simulink model "test_socket"  (Simulink 7.4)
settings: Solver=ode45  StartTime=0.0  StopTime=15.0  FixedStep=0.01  RelTol=1e-3
libraries: instrumentlib x2
settings Model: Creator=tasora  LastModifiedBy=tasora

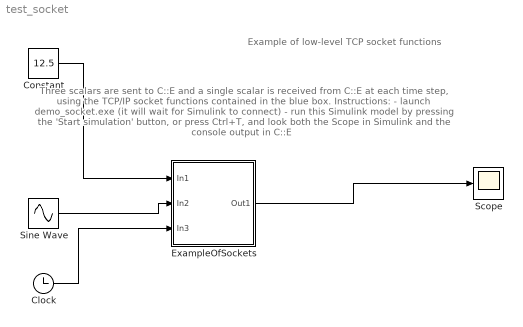
== system test_socket ==
  note: Three scalars are sent to C::E and a single scalar is received from C::E
      | at each time step, using the TCP/IP socket functions contained in the blue box.
      | Instructions:
      | - launch demo_socket.exe (it will wait for Simulink to connect)
      | - run this Simulink model by pressing the 'Start simulation' button, or press Ctrl+T,
      |   and look both the Scope in Simulink and the console output in C::E
  note: Example of low-level TCP socket functions
  Clock : Clock
      settings: Decimation=10
  Constant : Constant  Value=12.5  OutDataType=fixdt(1, 16)  OutScaling=2^0
  ExampleOfSockets : Subsystem  mask{com_step=0.2, tcp_data_size=1, host_name=localhost, tcp_port=50009, tcp_timeout=10}
      mask prompts: com_step "Communication step size"; tcp_data_size "Received data size (n. of scalars)"; host_name "TCP host name (ex. 'localhost', or 'www.myhost.com')"; tcp_port "TCP port (ex. 50007)"; tcp_timeout "TCP timeout (seconds)"
      mask init:
      | block_receive = [gcb, '/TCP Receive'];
      | set_param(block_receive, 'SampleTime', num2str(com_step));
      | set_param(block_receive, 'Host', host_name);
      | set_param(block_receive, 'Port', num2str(tcp_port));
      | set_param(block_receive, 'DataSize', num2str(tcp_data_size));
      | set_param(block_receive, 'Timeout', num2str(tcp_timeout));
      | block_send = [gcb, '/TCP Send'];
      | set_param(block_send, 'Host', host_name);
      | set_param(block_send, 'Port', num2str(tcp_port));
      mask Display: disp('C::E socket IO')
  Scope : Scope
  Sine Wave : Sin  Amplitude=5  Bias=0  Frequency=0.5  Phase=0  Samples=10  SampleTime=0  Offset=0
  wires:
  Constant/1 -> ExampleOfSockets/1(In1)
  Sine Wave/1 -> ExampleOfSockets/2(In2)
  Clock/1 -> ExampleOfSockets/3(In3)
  ExampleOfSockets/1(Out1) -> Scope/1

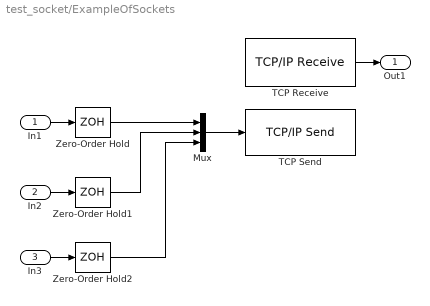
== system test_socket/ExampleOfSockets ==
  In1 : Inport
  In2 : Inport  Port=2
  In3 : Inport  Port=3
  Mux : Mux  Inputs=3
  TCP Receive : instrumentlib/TCP//IP Receive  Priority=1  DialogController=instrumentcreatedialog  DialogControllerArgs=DataTag0  Host=localhost  Port=50009  DataSize=1  EnableBlockingMode=on  Timeout=10  SampleTime=0.2  DataType=double  ByteOrder=LittleEndian
  TCP Send : instrumentlib/TCP//IP Send  Priority=2  DialogController=instrumentcreatedialog  DialogControllerArgs=DataTag1  Host=localhost  Port=50009  EnableBlockingMode=off  Timeout=10  ByteOrder=LittleEndian
  Zero-Order Hold : ZeroOrderHold  SampleTime=com_step
  Zero-Order Hold1 : ZeroOrderHold  SampleTime=com_step
  Zero-Order Hold2 : ZeroOrderHold  SampleTime=com_step
  Out1 : Outport
  wires:
  Zero-Order Hold/1 -> Mux/1
  Zero-Order Hold1/1 -> Mux/2
  Mux/1 -> TCP Send/1
  Zero-Order Hold2/1 -> Mux/3
  TCP Receive/1 -> Out1/1
  In1/1 -> Zero-Order Hold/1
  In2/1 -> Zero-Order Hold1/1
  In3/1 -> Zero-Order Hold2/1
